simulink model "sfcndemo_ada_matrix_gain"  (Simulink 6.0)
settings: Solver=FixedStepDiscrete  StartTime=0.0  StopTime=10  FixedStep=0.1  RelTol=1e-3
settings Model: Creator=The MathWorks Inc.  LastModifiedBy=batserve  ExtModeTrigMode=oneshot  ExtModeArmWhenConnect=off  ExtModeAutoUpdateStatusClock=off
settings DataIOCC: LimitDataPoints=off  StateSaveName=x  TimeSaveName=t  OutputSaveName=y
settings OptimizationCC: BlockReduction=off  BooleanDataType=off  InlineInvariantSignals=off
settings DebuggingCC: ConsistencyChecking=error  ArrayBoundsChecking=error  CheckExecutionContextPreStartOutputMsg=on  CheckExecutionContextRuntimeOutputMsg=on  SolverPrmCheckMsg=none
settings HardwareCC: TargetUnknown=on
settings RTWCC: SystemTargetFile=rt_ada_sim.tlc  MakeCommand=make_rtw -ada=gnat3.12a2 -v  TemplateMakefile=gnat_sim.tmf  RetainRTWFile=on  ProcessScript=rt_ada_sim_make_rtw_hook
settings STFCustomTargetCC: TargetFcnLib=ansi_tfl_tmw.mat  GenFloatMathFcnCalls=ANSI_C  ModelReferenceCompliant=off  CombineOutputUpdateFcns=on  MatFileLogging=on  SystemTargetFile=rt_ada_sim.tlc

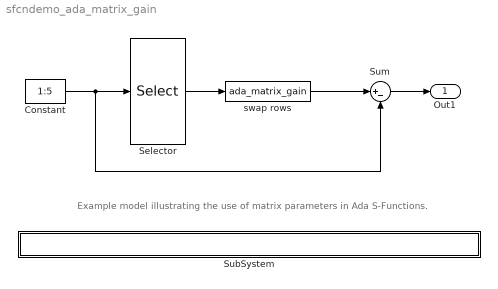
== system sfcndemo_ada_matrix_gain ==
  note: Example model illustrating the use of matrix parameters in Ada S-Functions.
  Constant : Constant  Value=1:5
  Selector : Selector  Elements=[2 5 1 3 4]  InputPortWidth=5
  SubSystem : Subsystem  PropExecContextAcrossSSBoundary=on
      settings: OpenFcn=evalin('base','edit(fullfile(matlabroot,''simulink'',''ada'',''examples'',''matrix_gain'',''matrix_gain.adb''))')
      mask Display: disp('matlabroot\simulink\ada\examples\matrix_gain\matrix_gain.adb');
  Sum : Sum  Inputs=|+-  SaturateOnIntegerOverflow=on  InputSameDT=on
  swap rows : S-Function  FunctionName=ada_matrix_gain  Parameters=[0 0 1 0 0; 1 0 0 0 0; 0 0 0 1 0; 0 0 0 0 1; 0 1 0 0 0]
  Out1 : Outport
  wires:
  Constant/1 -> Selector/1, Sum/2
  Selector/1 -> swap rows/1
  swap rows/1 -> Sum/1
  Sum/1 -> Out1/1

== system sfcndemo_ada_matrix_gain/SubSystem ==
